simulink model "MassSpringDamperSolution"  (R2025a)
settings: Solver=VariableStepAuto  StartTime=0.0  StopTime=10.0  RelTol=1e-3
undefined symbols (not defined in the file): b, F, k, M
settings Model: Creator=Pablo  LastModifiedBy=Pablo

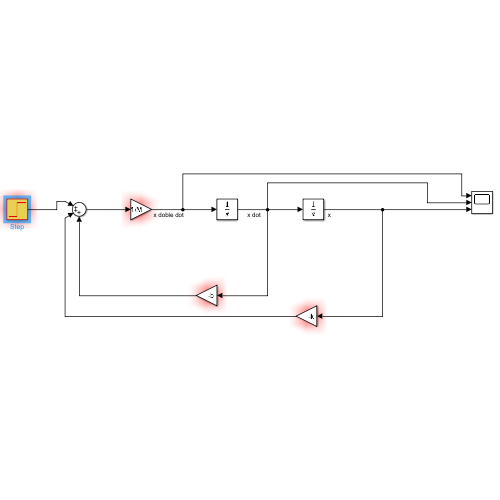
[thumbnail: Simulink's stored preview of the top-level diagram]
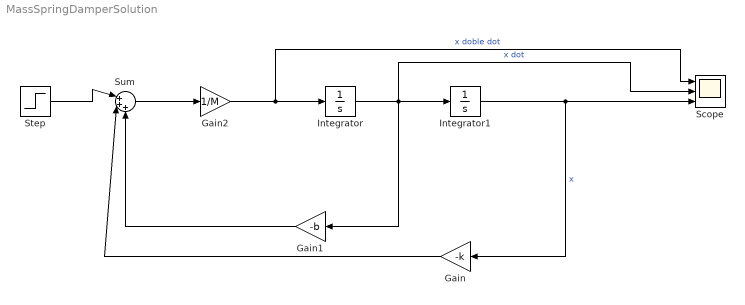
== system MassSpringDamperSolution ==
  Gain : Gain  Gain=-k
  Gain1 : Gain  Gain=-b
  Gain2 : Gain  Gain=1/M
  Integrator : Integrator
  Integrator1 : Integrator
  Scope : Scope  NumInputPorts=3
      settings: ActiveDisplayYMinimum=-1.1526991715970936  ActiveDisplayYMaximum=1.2391887968441215
  Step : Step  Time=F  After=F  SampleTime=0
  Sum : Sum  Inputs=|+++
  wires:
  Step/1 -> Sum/1
  Gain1/1 -> Sum/3
  Gain/1 -> Sum/2
  Sum/1 -> Gain2/1
  Gain2/1 -> Scope/1, Integrator/1  "x doble dot"
  Integrator/1 -> Gain1/1, Scope/2, Integrator1/1  "x dot"
  Integrator1/1 -> Gain/1, Scope/3  "x"
